simulink model "demo"  (R2013a)
settings: Solver=ode45  StartTime=0.0  StopTime=10.0  RelTol=1e-3
settings Model: Creator=Arnaud  LastModifiedBy=Arnaud

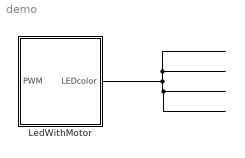
== system demo ==
  LedWithMotor : Subsystem
  wires:
  ? -> LedWithMotor/1(PWM)
  LedWithMotor/1(LEDcolor) -> ?
  ? -> ?

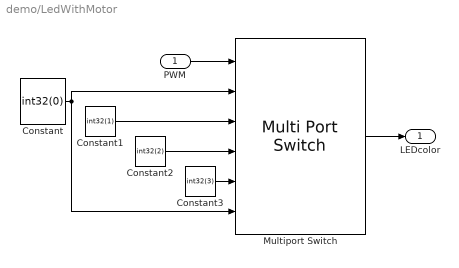
== system demo/LedWithMotor ==
  PWM : Inport
  Constant : Constant  Value=int32(0)
  Constant1 : Constant  Value=int32(1)
  Constant2 : Constant  Value=int32(2)
  Constant3 : Constant  Value=int32(3)
  Multiport Switch : MultiPortSwitch  DataPortOrder=Specify indices  Inputs=4  DataPortIndices={[0.0:25.0],[26:50],[51:75],[76:100]}  DataPortForDefault=Additional data port  OutDataTypeStr=int32
  LEDcolor : Outport
  wires:
  Constant/1 -> Multiport Switch/2, Multiport Switch/6
  PWM/1 -> Multiport Switch/1
  Multiport Switch/1 -> LEDcolor/1
  Constant1/1 -> Multiport Switch/3
  Constant2/1 -> Multiport Switch/4
  Constant3/1 -> Multiport Switch/5
